simulink model "SixDof"  (R2023a)
settings: Solver=VariableStepAuto  StartTime=0.0  StopTime=60  RelTol=1e-3
values from neighbouring files (symbols this model uses):
  b = 9.144    [FS.m]
  c = 3.45    [FS.m]
  delta_r = 0    [FS.m]
  deltalef = 0    [FS.m]
  deltaSB = 0    [FS.m]
  F16_LookupTables =     [F16_LookupTables.mat]
  g = 9.80665    [FS.m]
  Ixx = 12875    [FS.m]
  Ixz = 1331    [FS.m]
  Iyy = 75674    [FS.m]
  Izz = 85552    [FS.m]
  mass = 9300    [FS.m]
  S = 27.88    [FS.m]
undefined symbols (not defined in the file or in its folder): Earth, WGS84
libraries: coeff x6, simulink_extras x4, shared6dof x1, aerolibtransform2 x1, aerolibfltsims x1, AtmosferModel x1, aerolibasang x1, simulink x1, sharedtransform x1, propulsive x1, uavutilslib x1
(part 1 of 2)
settings Model: Creator=User  LastModifiedBy=User
settings SolverCC: ZeroCrossAlgorithm=Adaptive
settings DebuggingCC: MaskedZcDiagnostic=none  IgnoredZcDiagnostic=none

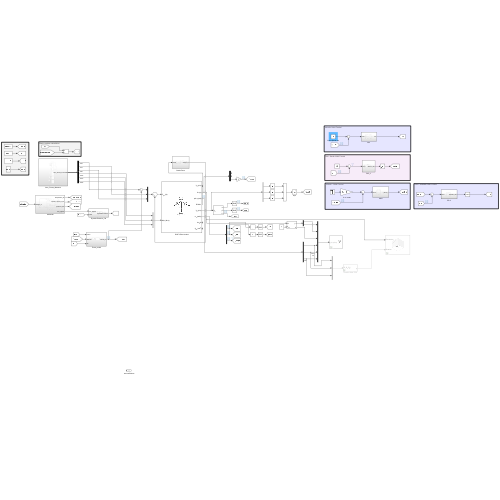
[thumbnail: Simulink's stored preview of the top-level diagram]
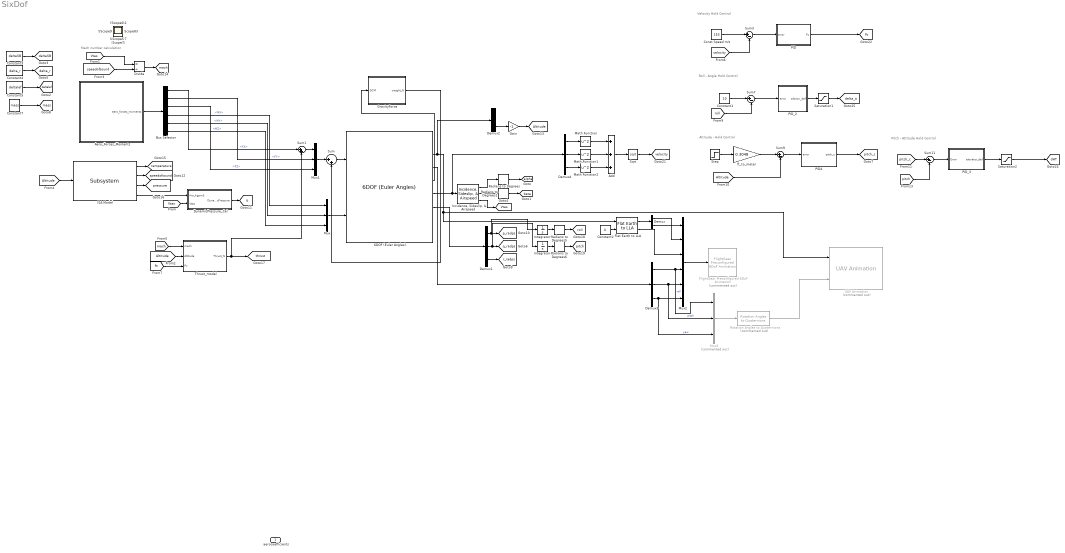
== system SixDof ==
  note: Altitude - Hold Control
  note: Pitch - Attitude Hold Control
  note: Roll - Angle Hold Control
  note: Velocity Hold Control
  note: Mach number calculation
  6DOF (Euler Angles) : shared6dof/6DOF (Euler Angles)  units=Metric (MKS)  mtype=Fixed  rep=Euler Angles  xme_0=[0 0 -3048]  Vm_0=[0 153 0]  eul_0=[0 0 0]  pm_0=[0 0 0]  mass_0=mass  mass_e=0.5  mass_f=2.0  inertia=[Ixx 0 Ixz; 0 Iyy 0; 0 0 Izz]  inertia_e=eye(3)  inertia_f=2*eye(3)  k_quat=1.0  vre_flag=on  abi_flag=off  aMode=0  xme_statename=''  Vm_statename=''  eul_statename=''  quat_statename=''  pm_statename=''  mass_statename=''
  Add : Sum  Inputs=+++
  Aero_Forces_Moments : Subsystem
  Bus Selector : BusSelector  OutputSignals=FX,FY,FZ,MX,MY,MZ
  Const Speed m/s : Constant  Value=153
  Constant1 : Constant  Value=10
  Constant2 : Constant  Value=0
  Constant3 : Constant  Value=deltaSB
  Constant4 : Constant  Value=delta_r
  Constant5 : Constant  Value=deltalef
  Constant7 : Constant  Value=mass
  Demux : Demux  Outputs=2
  Demux{1..4} (4 alike) : Demux  Outputs=3
  Divide : Product  Inputs=*/
  DynamicPressure_Cal : Subsystem
  Flat Earth to LLA : aerolibtransform2/Flat Earth to LLA  units=Metric (MKS)  ptype=Earth (WGS84)  F=1/298.257223563  R=6378137  refPosPort=off  LL0=[0 10]  psi=0
  FlightGear Preconfigured 6DoF Animation : aerolibfltsims/FlightGear Preconfigured 6DoF Animation  Commented=on  xFlightGearVersion=v2019.1  DestinationIpAddress=127.0.0.1  DestinationPort=5502  SampleTime=1/30  packetVersion=24
  Gain : Gain  Gain=-1
  GravityForce : Subsystem
  ISA Model : AtmosferModel/Subsystem  SystemSampleTime=-1  VariantActivationTime=update diagram  Latency=0  AutoFrameSizeCalculation=off
  "Incidence, Sideslip, & Airspeed" : aerolibasang/Incidence, Sideslip, & Airspeed
  Integrator2 : Integrator
  Integrator4 : Integrator
  Math Function : Math  Operator=square
  Math Function1 : Math  Operator=square
  Math Function2 : Math  Operator=square
  Mux : Mux  Inputs=3
  Mux1 : Mux  Inputs=3
  Mux2 : Mux  Inputs=6
  Mux3 : Mux  Commented=on  Inputs=3
  "PID " : Subsystem
  PID4 : Subsystem
  PID_2 : Subsystem
  PID_3 : Subsystem
  Radians to Degrees{,1,5..6} (4 alike) : simulink_extras/Transformations/Radians to Degrees
  Rotation Angles to Quaternions : sharedtransform/Rotation Angles to Quaternions  Commented=on  rotationOrder=ZYX  aMode=aMode
  Saturation1 : Saturate  UpperLimit=20  LowerLimit=-20
  Saturation2 : Saturate  UpperLimit=20  LowerLimit=-20  LinearizeAsGain=off  ZeroCross=off
  Sqrt : Sqrt  IntermediateResultsDataTypeStr=double
  Step : Step  Time=30  Before=11000  After=9900  SampleTime=0
  Sum : Sum  Inputs=|++
  Sum1 : Sum  Inputs=|++
  Sum{3,7,9,11} (4 alike) : Sum  Inputs=|+-
  Thrust_model : Subsystem
  UAV Animation : uavutilslib/UAV Animation  Commented=on  UAVType=FixedWing  UAVSize=1  InertialZDirection=Down  SampleTime=-1
  ft_to_meter : Gain  Gain=0.3048
  aerocoefficients : Outport
  Scope{,1..44} (45 alike) : Scope
  tag scope: Altitude=global, Pc=global, Vtas=global, alpha=global, beta=global, dHT=global, deltaSB=global, delta_a=global, delta_r=global, deltalef=global, mach=global, mass=global, p_radps=global, pitch=global, pitch_c=global, pressure=global, q=global, q_radps=global, r_radps=global, roll=global, speedofsound=global, temperature=global, thrust=global, velocity=global
  wires:
  [speedofsound] -> Divide/2
  [Vtas] -> Divide/1
  Demux1/1 -> Integrator2/1, [p_radps]
  Demux1/2 -> Integrator4/1, [q_radps]
  Demux1/3 -> [r_radps]
  6DOF (Euler Angles)/6 -> Demux1/1
  Aero_Forces_Moments/1(aero_forces_moments) -> Bus Selector/1
  Mux/1 -> 6DOF (Euler Angles)/2
  Constant3/1 -> [deltaSB]
  Constant4/1 -> [delta_r]
  Constant5/1 -> [deltalef]
  Constant7/1 -> [mass]
  6DOF (Euler Angles)/5 -> Demux4/1, "Incidence, Sideslip, & Airspeed"/1
  "Incidence, Sideslip, & Airspeed"/1 -> Radians to Degrees/1
  "Incidence, Sideslip, & Airspeed"/2 -> Radians to Degrees1/1
  "Incidence, Sideslip, & Airspeed"/3 -> [Vtas]
  Bus Selector/2 -> Mux1/2  "<FY>"
  Bus Selector/4 -> Mux/1  "<MX>"
  Bus Selector/5 -> Mux/2  "<MY>"
  Bus Selector/6 -> Mux/3  "<MZ>"
  Bus Selector/3 -> Mux1/3  "<FZ>"
  Mux1/1 -> Sum/1
  Sum/1 -> 6DOF (Euler Angles)/1
  6DOF (Euler Angles)/2 -> Demux2/1, Flat Earth to LLA/1, UAV Animation/1
  Radians to Degrees1/1 -> [beta]
  Radians to Degrees/1 -> [alpha]
  6DOF (Euler Angles)/4 -> GravityForce/1(DCM)
  GravityForce/1(weight_N) -> Sum/2
  DynamicPressure_Cal/1(DynamicPressure) -> [q]
  [Vtas] -> DynamicPressure_Cal/2(Vtas)
  Divide/1 -> [mach]
  Sum1/1 -> Mux1/1
  Bus Selector/1 -> Sum1/1  "<FX>"
  Thrust_model/1(Thrust_N) -> Sum1/2, [thrust]
  [mach] -> Thrust_model/1(mach)
  [Altitude] -> Thrust_model/2(Altitude)
  [Altitude] -> ISA Model/1
  ISA Model/3 -> [pressure]
  ISA Model/2 -> [speedofsound]
  ISA Model/1 -> [temperature]
  ISA Model/4 -> DynamicPressure_Cal/1(rho_kgpm3)
  Gain/1 -> [Altitude]
  6DOF (Euler Angles)/3 -> Demux3/1
  Demux4/1 -> Math Function/1
  Demux4/3 -> Math Function2/1
  Demux4/2 -> Math Function1/1
  Math Function/1 -> Add/1
  Math Function1/1 -> Add/2
  Math Function2/1 -> Add/3
  Add/1 -> Sqrt/1
  Sqrt/1 -> [velocity]
  [velocity] -> Sum3/2
  Const Speed m/s/1 -> Sum3/1
  [Pc] -> Thrust_model/3(Pc)
  [roll] -> Sum7/2
  Integrator2/1 -> Radians to Degrees5/1
  Radians to Degrees5/1 -> [roll]
  Integrator4/1 -> Radians to Degrees6/1
  Radians to Degrees6/1 -> [pitch]
  [Altitude] -> Sum9/2
  [pitch] -> Sum11/2
  Sum3/1 -> "PID "/1(error)
  "PID "/1(Pc) -> [Pc]
  Sum7/1 -> PID_2/1(error)
  PID_2/1(aileron_def) -> Saturation1/1
  Sum11/1 -> PID_3/1(Error)
  PID_3/1(elevator_def) -> Saturation2/1
  Saturation1/1 -> [delta_a]
  Mux2/1 -> FlightGear Preconfigured 6DoF Animation/1
  Flat Earth to LLA/1 -> Demux/1
  Demux/2 -> Mux2/1
  Demux/1 -> Mux2/2
  Constant2/1 -> Flat Earth to LLA/2
  Flat Earth to LLA/2 -> Mux2/3
  Demux3/1 -> Mux3/1, Mux2/4  "roll"
  Demux3/2 -> Mux3/2, Mux2/5  "pitch"
  Demux3/3 -> Mux3/3, Mux2/6  "yaw"
  Constant1/1 -> Sum7/1
  Step/1 -> ft_to_meter/1
  ft_to_meter/1 -> Sum9/1
  Saturation2/1 -> [dHT]
  Rotation Angles to Quaternions/1 -> UAV Animation/2
  Mux3/1 -> Rotation Angles to Quaternions/1
  [pitch_c] -> Sum11/1
  Demux2/3 -> Gain/1
  Sum9/1 -> PID4/1(error)
  PID4/1(pitch_c) -> [pitch_c]

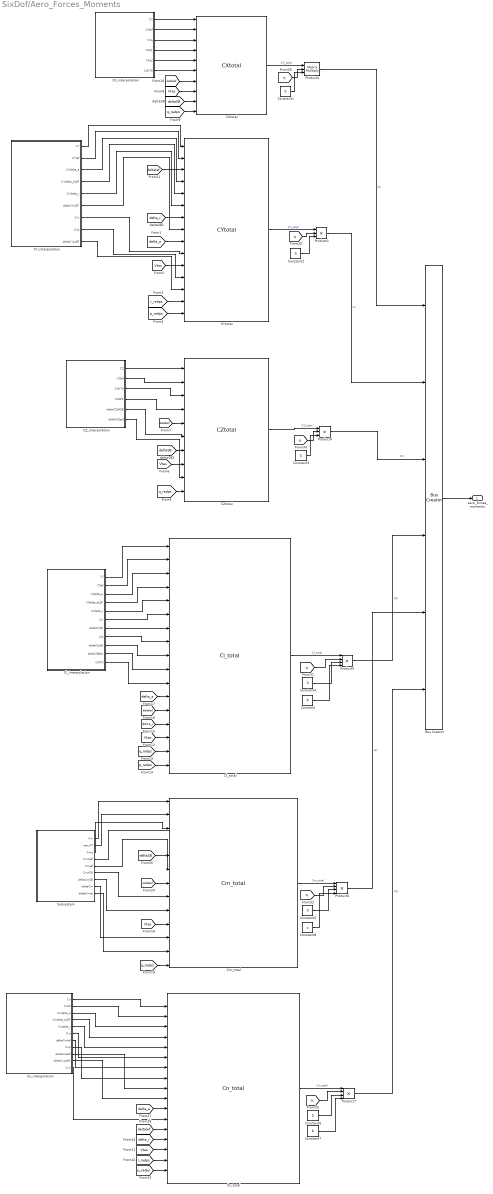
== system SixDof/Aero_Forces_Moments ==
  Bus Creator : BusCreator  Inputs=6
  CX_interpolation : Subsystem
  CXtotal : coeff/CXtotal  SystemSampleTime=-1  VariantActivationTime=update diagram  Latency=0  AutoFrameSizeCalculation=off
  CY_interpolation : Subsystem
  CYtotal : coeff/CYtotal  SystemSampleTime=-1  VariantActivationTime=update diagram  Latency=0  AutoFrameSizeCalculation=off
  CZ_interpolation : Subsystem
  CZtotal : coeff/CZtotal  SystemSampleTime=-1  VariantActivationTime=update diagram  Latency=0  AutoFrameSizeCalculation=off
  Cl_interpolation : Subsystem
  Cl_total : coeff/Cl_total  SystemSampleTime=-1  VariantActivationTime=update diagram  Latency=0  AutoFrameSizeCalculation=off
  Cm_total : coeff/Cm_total  SystemSampleTime=-1  VariantActivationTime=update diagram  Latency=0  AutoFrameSizeCalculation=off
  Cn_interpolation : Subsystem
  Cn_total : coeff/Cn_total  SystemSampleTime=-1  VariantActivationTime=update diagram  Latency=0  AutoFrameSizeCalculation=off
  Constant : Constant  Value=b
  Constant{1..6} (6 alike) : Constant  Value=S
  Constant7 : Constant  Value=b
  Constant8 : Constant  Value=c
  Product2 : Product  Inputs=3  Multiplication=Matrix(*)
  Product3 : Product  Inputs=3
  Product4 : Product  Inputs=3
  Product5 : Product  Inputs=4
  Product6 : Product  Inputs=4
  Product7 : Product  Inputs=4
  Subsystem : Subsystem
  aero_forces_moments : Outport
  wires:
  [p_radps] -> Cl_total/17
  CY_interpolation/3(CYdelta_a) -> CYtotal/4
  Cn_interpolation/9(deltaCnplef) -> Cn_total/9
  Subsystem/9(deltaCmds) -> Cm_total/12
  CZ_interpolation/1(CZ) -> CZtotal/1
  [deltalef] -> Cl_total/13
  [Vtas] -> Cm_total/10
  CX_interpolation/4(CXq1) -> CXtotal/4
  [deltalef] -> CXtotal/7
  [Vtas] -> CXtotal/8
  [p_radps] -> CYtotal/15
  Cl_interpolation/2(Cllef) -> Cl_total/2
  CZ_interpolation/5(deltaCZlefSB) -> CZtotal/6
  Cl_interpolation/4(Cldelta_aLEF) -> Cl_total/4
  Cl_interpolation/3(Cldelta_a) -> Cl_total/3
  CX_interpolation/1(CX) -> CXtotal/1
  Subsystem/4(Cmqlef) -> Cm_total/4
  CX_interpolation/2(CXlef) -> CXtotal/2
  CY_interpolation/8(CYp) -> CYtotal/12
  [Vtas] -> Cn_total/15
  Subsystem/3(Cmq) -> Cm_total/3
  Cl_interpolation/10(deltaClBeta) -> Cl_total/10
  Subsystem/7(deltaCmSB) -> Cm_total/9
  CX_interpolation/3(CXq) -> CXtotal/3
  Cn_interpolation/2(Cnlef) -> Cn_total/2
  [deltaSB] -> CXtotal/9
  CZ_interpolation/4(CZlef1) -> CZtotal/4
  CY_interpolation/1(CY) -> CYtotal/1
  CX_interpolation/5(CXq2) -> CXtotal/5
  CX_interpolation/6(CXHT0) -> CXtotal/6
  [r_radps] -> Cn_total/16
  Subsystem/5(Cmlef) -> Cm_total/6
  CY_interpolation/2(CYlef) -> CYtotal/2
  CY_interpolation/4(CYdelta_aLEF) -> CYtotal/5
  [q_radps] -> Cl_total/16
  CZ_interpolation/3(CZHT0) -> CZtotal/3
  [deltalef] -> CYtotal/3
  Cn_interpolation/3(Cndelta_a) -> Cn_total/3
  [Vtas] -> CYtotal/11
  Subsystem/8(deltaCm) -> Cm_total/11
  Cl_interpolation/9(deltaClplef) -> Cl_total/9
  [delta_a] -> CYtotal/9
  Cl_interpolation/6(Clr) -> Cl_total/6
  [deltaSB] -> CZtotal/7
  CY_interpolation/6(deltaCYrLEF) -> CYtotal/8
  CZ_interpolation/2(CZlef) -> CZtotal/2
  [deltalef] -> Cm_total/7
  [delta_r] -> CYtotal/7
  Cl_interpolation/7(deltaClrlef) -> Cl_total/7
  CY_interpolation/9(deltaCYpLEF) -> CYtotal/13
  CZ_interpolation/6(deltaCZlqef) -> CZtotal/9
  [Vtas] -> CZtotal/8
  [Vtas] -> Cl_total/15
  Cn_interpolation/7(deltaCnrlef) -> Cn_total/7
  Subsystem/1(Cm) -> Cm_total/1
  Cl_interpolation/11(ClHT0) -> Cl_total/11
  [r_radps] -> CYtotal/14
  Cl_interpolation/8(Clp) -> Cl_total/8
  [q_radps] -> CZtotal/10
  [deltaSB] -> Cm_total/5
  Cl_interpolation/1(Cl) -> Cl_total/1
  [p_radps] -> Cn_total/17
  [q_radps] -> Cm_total/13
  Subsystem/6(CmHT0) -> Cm_total/8
  Cn_interpolation/6(Cnr) -> Cn_total/6
  Cn_interpolation/1(Cn) -> Cn_total/1
  CY_interpolation/7(CYr) -> CYtotal/10
  [deltalef] -> CZtotal/5
  Cn_interpolation/5(Cndelta_r) -> Cn_total/5
  Cn_interpolation/8(Cnp) -> Cn_total/8
  CY_interpolation/5(CYdelta_r) -> CYtotal/6
  Subsystem/2(eta_HT) -> Cm_total/2
  [q_radps] -> CXtotal/10
  Cl_interpolation/5(Cldelta_r) -> Cl_total/5
  Cn_interpolation/11(Cn1) -> Cn_total/12
  Cn_interpolation/4(Cndelta_aLEF) -> Cn_total/4
  [deltalef] -> Cn_total/13
  Cn_interpolation/10(deltaCnplef1) -> Cn_total/10
  Constant1/1 -> Product2/3
  [q] -> Product2/2
  CXtotal/1 -> Product2/1  "CX_total"
  Constant2/1 -> Product3/3
  [q] -> Product3/2
  CYtotal/1 -> Product3/1  "CY_total"
  Constant3/1 -> Product4/3
  [q] -> Product4/2
  CZtotal/1 -> Product4/1  "CZ_total"
  Constant4/1 -> Product5/3
  [q] -> Product5/2
  Cl_total/1 -> Product5/1  "Cl_total"
  Constant5/1 -> Product6/3
  [q] -> Product6/2
  Cm_total/1 -> Product6/1  "Cm_total"
  Constant6/1 -> Product7/3
  [q] -> Product7/2
  Cn_total/1 -> Product7/1  "Cn_total"
  Product2/1 -> Bus Creator/1  "FX"
  Product3/1 -> Bus Creator/2  "FY"
  Product4/1 -> Bus Creator/3  "FZ"
  Product5/1 -> Bus Creator/4  "MX"
  Product6/1 -> Bus Creator/5  "MY"
  Product7/1 -> Bus Creator/6  "MZ"
  Bus Creator/1 -> aero_forces_moments/1
  Constant/1 -> Product5/4
  Constant8/1 -> Product6/4
  Constant7/1 -> Product7/4
  [delta_a] -> Cl_total/12
  [delta_r] -> Cl_total/14
  [delta_a] -> Cn_total/11
  [delta_r] -> Cn_total/14

== system SixDof/DynamicPressure_Cal ==
  rho_kgpm3 : Inport
  Vtas : Inport  Port=2
  Gain : Gain  Gain=0.5
  Math Function : Math  Operator=square
  Product : Product
  DynamicPressure : Outport
  wires:
  Math Function/1 -> Gain/1
  Gain/1 -> Product/1
  rho_kgpm3/1 -> Product/2
  Product/1 -> DynamicPressure/1
  Vtas/1 -> Math Function/1

== system SixDof/GravityForce ==
  DCM : Inport
  Constant1 : Constant  Value=0
  Mux2 : Mux  Inputs=3
  Product1 : Product  Multiplication=Matrix(*)
  g_mps2 : Gain  Gain=g
  weight_N : Outport
  wires:
  Constant1/1 -> Mux2/1, Mux2/2
  Mux2/1 -> Product1/2
  g_mps2/1 -> Mux2/3  "weight_N"
  [mass] -> g_mps2/1
  Product1/1 -> weight_N/1  "weight_N"
  DCM/1 -> Product1/1

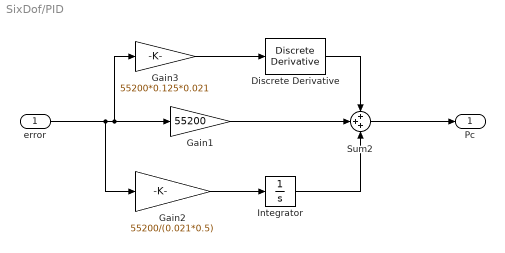
== system SixDof/PID  ==
  error : Inport
  Discrete Derivative : simulink/Discrete/Discrete Derivative  gainval=1.0  ICPrevScaledInput=0.0  OutMin=[]  OutMax=[]  OutDataType=fixdt(1, 16)  OutScaling=2^-10  DoSatur=off
  Gain1 : Gain  Gain=55200
  Gain2 : Gain  Gain=55200/(0.021*0.5)
  Gain3 : Gain  Gain=55200*0.125*0.021
  Integrator : Integrator
  Sum2 : Sum  Inputs=+++
  Pc : Outport
  wires:
  Gain3/1 -> Discrete Derivative/1
  Discrete Derivative/1 -> Sum2/1
  Integrator/1 -> Sum2/3
  Gain2/1 -> Integrator/1
  error/1 -> Gain2/1, Gain3/1, Gain1/1
  Gain1/1 -> Sum2/2
  Sum2/1 -> Pc/1

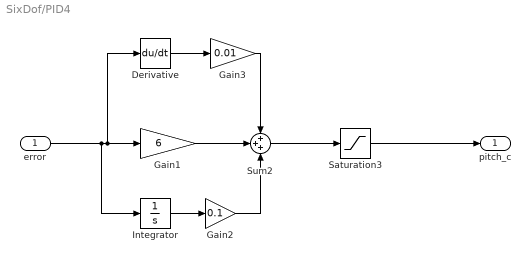
== system SixDof/PID4 ==
  error : Inport
  Derivative : Derivative
  Gain1 : Gain  Gain=6
  Gain2 : Gain  Gain=0.1
  Gain3 : Gain  Gain=0.01
  Integrator : Integrator
  Saturation3 : Saturate  UpperLimit=5  LowerLimit=-5
  Sum2 : Sum  Inputs=+++
  pitch_c : Outport
  wires:
  Gain1/1 -> Sum2/2
  error/1 -> Integrator/1, Derivative/1, Gain1/1
  Gain3/1 -> Sum2/1
  Derivative/1 -> Gain3/1
  Integrator/1 -> Gain2/1
  Gain2/1 -> Sum2/3
  Sum2/1 -> Saturation3/1
  Saturation3/1 -> pitch_c/1

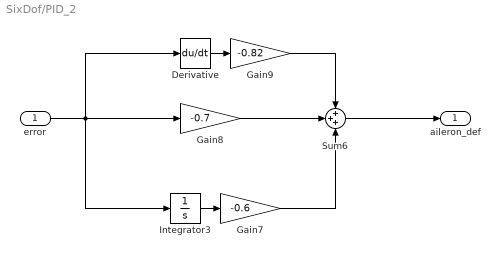
== system SixDof/PID_2 ==
  error : Inport
  Derivative : Derivative
  Gain7 : Gain  Gain=-0.6
  Gain8 : Gain  Gain=-0.7
  Gain9 : Gain  Gain=-0.82
  Integrator3 : Integrator
  Sum6 : Sum  Inputs=+++
  aileron_def : Outport
  wires:
  Gain7/1 -> Sum6/3
  error/1 -> Derivative/1, Integrator3/1, Gain8/1
  Gain8/1 -> Sum6/2
  Sum6/1 -> aileron_def/1
  Gain9/1 -> Sum6/1
  Integrator3/1 -> Gain7/1
  Derivative/1 -> Gain9/1

== system SixDof/PID_3 ==
  Error : Inport
  Derivative2 : Derivative
  Gain13 : Gain  Gain=-1.89
  Gain14 : Gain  Gain=-8
  Gain15 : Gain  Gain=-6
  Integrator6 : Integrator
  Sum10 : Sum  Inputs=+++
  elevator_def : Outport
  wires:
  Error/1 -> Integrator6/1, Derivative2/1, Gain14/1
  Gain15/1 -> Sum10/1
  Gain14/1 -> Sum10/2
  Derivative2/1 -> Gain15/1
  Integrator6/1 -> Gain13/1
  Gain13/1 -> Sum10/3
  Sum10/1 -> elevator_def/1

== system SixDof/Thrust_model ==
  mach : Inport
  Altitude : Inport  Port=2
  Pc : Inport  Port=3
  Propulsion : propulsive/Propulsive Force  SystemSampleTime=-1  VariantActivationTime=update diagram  Latency=0  AutoFrameSizeCalculation=off
  Thrust_interpolation : Subsystem
  ibstoN : Gain  Gain=4.4482216153
  meter_to_ft : Gain  Gain=3.28
  Thrust_N : Outport
  wires:
  ibstoN/1 -> Thrust_N/1
  Thrust_interpolation/3(max) -> Propulsion/3
  Thrust_interpolation/2(mil) -> Propulsion/2
  Thrust_interpolation/1(idle) -> Propulsion/1
  Propulsion/1 -> ibstoN/1
  meter_to_ft/1 -> Thrust_interpolation/2(altitude_ft)
  mach/1 -> Thrust_interpolation/1(mach)
  Altitude/1 -> meter_to_ft/1
  Pc/1 -> Propulsion/4

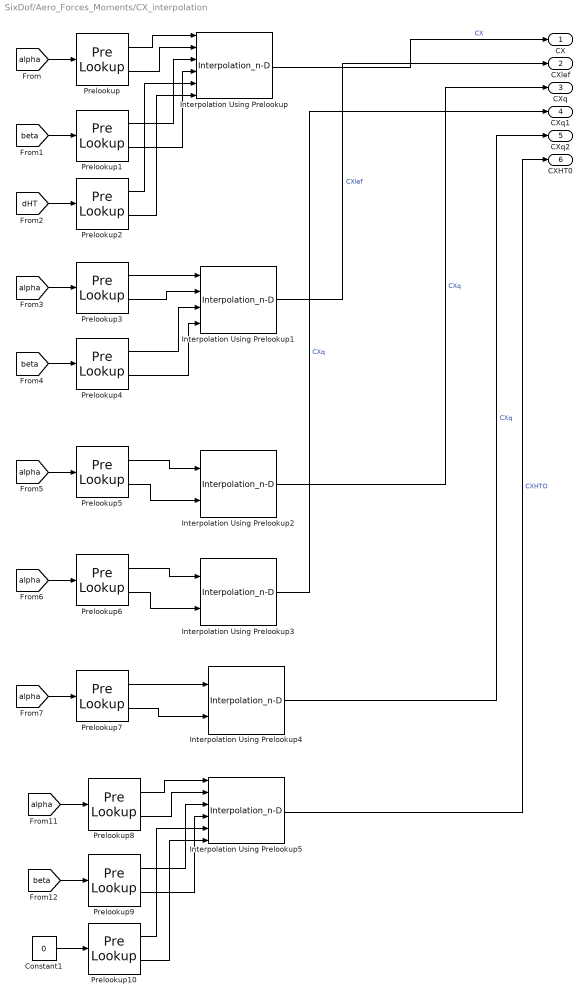
== system SixDof/Aero_Forces_Moments/CX_interpolation ==
  Constant1 : Constant  Value=0
  Interpolation Using Prelookup : Interpolation_n-D  NumberOfTableDimensions=3  Table=F16_LookupTables.aero.data.CX.CX  InternalRulePriority=Speed
      settings: InputPortMap=u0,u1,u2,u3,u4,u5
  Interpolation Using Prelookup1 : Interpolation_n-D  Table=F16_LookupTables.aero.data.CX.CXlef  InternalRulePriority=Speed
  Interpolation Using Prelookup2 : Interpolation_n-D  NumberOfTableDimensions=1  Table=F16_LookupTables.aero.data.CX.CXq  InternalRulePriority=Speed
      settings: InputPortMap=u0,u1
  Interpolation Using Prelookup3 : Interpolation_n-D  NumberOfTableDimensions=1  Table=F16_LookupTables.aero.data.CX.deltaCXqlef  InternalRulePriority=Speed
      settings: InputPortMap=u0,u1
  Interpolation Using Prelookup4 : Interpolation_n-D  NumberOfTableDimensions=1  Table=F16_LookupTables.aero.data.CX.deltaCXSB  InternalRulePriority=Speed
      settings: InputPortMap=u0,u1
  Interpolation Using Prelookup5 : Interpolation_n-D  NumberOfTableDimensions=3  Table=F16_LookupTables.aero.data.CX.CX  InternalRulePriority=Speed
      settings: InputPortMap=u0,u1,u2,u3,u4,u5
  Prelookup : PreLookup  BreakpointsData=F16_LookupTables.aero.inputs.CX.CX.alpha  ExtrapMethod=Linear
  Prelookup1 : PreLookup  BreakpointsData=F16_LookupTables.aero.inputs.CX.CX.beta  ExtrapMethod=Linear
  Prelookup10 : PreLookup  BreakpointsData=F16_LookupTables.aero.inputs.CX.CX.dHT  ExtrapMethod=Linear
  Prelookup2 : PreLookup  BreakpointsData=F16_LookupTables.aero.inputs.CX.CX.dHT  ExtrapMethod=Linear
  Prelookup3 : PreLookup  BreakpointsData=F16_LookupTables.aero.inputs.CX.CXlef.alpha  ExtrapMethod=Linear
  Prelookup4 : PreLookup  BreakpointsData=F16_LookupTables.aero.inputs.CX.CXlef.beta  ExtrapMethod=Linear
  Prelookup5 : PreLookup  BreakpointsData=F16_LookupTables.aero.inputs.CX.CXq.alpha  ExtrapMethod=Linear
  Prelookup6 : PreLookup  BreakpointsData=F16_LookupTables.aero.inputs.CX.deltaCXqlef.alpha  ExtrapMethod=Linear
  Prelookup7 : PreLookup  BreakpointsData=F16_LookupTables.aero.inputs.CX.deltaCXSB.alpha  ExtrapMethod=Linear
  Prelookup8 : PreLookup  BreakpointsData=F16_LookupTables.aero.inputs.CX.CX.alpha  ExtrapMethod=Linear
  Prelookup9 : PreLookup  BreakpointsData=F16_LookupTables.aero.inputs.CX.CX.beta  ExtrapMethod=Linear
  CX : Outport
  CXlef : Outport  Port=2
  CXq : Outport  Port=3
  CXq1 : Outport  Port=4
  CXq2 : Outport  Port=5
  CXHT0 : Outport  Port=6
  wires:
  [dHT] -> Prelookup2/1
  [beta] -> Prelookup9/1
  Prelookup4/1 -> Interpolation Using Prelookup1/3
  Constant1/1 -> Prelookup10/1
  Prelookup10/1 -> Interpolation Using Prelookup5/5
  [alpha] -> Prelookup3/1
  Prelookup1/1 -> Interpolation Using Prelookup/3
  [alpha] -> Prelookup5/1
  Prelookup10/2 -> Interpolation Using Prelookup5/6
  [alpha] -> Prelookup6/1
  Prelookup8/1 -> Interpolation Using Prelookup5/1
  Prelookup1/2 -> Interpolation Using Prelookup/4
  Interpolation Using Prelookup2/1 -> CXq/1  "CXq"
  [alpha] -> Prelookup8/1
  [beta] -> Prelookup4/1
  Interpolation Using Prelookup/1 -> CX/1  "CX"
  Interpolation Using Prelookup4/1 -> CXq2/1  "CXq"
  Prelookup9/2 -> Interpolation Using Prelookup5/4
  Prelookup/1 -> Interpolation Using Prelookup/1
  Prelookup/2 -> Interpolation Using Prelookup/2
  Prelookup3/1 -> Interpolation Using Prelookup1/1
  Prelookup4/2 -> Interpolation Using Prelookup1/4
  [alpha] -> Prelookup/1
  Prelookup5/2 -> Interpolation Using Prelookup2/2
  Prelookup3/2 -> Interpolation Using Prelookup1/2
  Prelookup2/1 -> Interpolation Using Prelookup/5
  Prelookup7/1 -> Interpolation Using Prelookup4/1
  [beta] -> Prelookup1/1
  Prelookup2/2 -> Interpolation Using Prelookup/6
  Prelookup9/1 -> Interpolation Using Prelookup5/3
  Prelookup6/2 -> Interpolation Using Prelookup3/2
  Prelookup6/1 -> Interpolation Using Prelookup3/1
  [alpha] -> Prelookup7/1
  Prelookup7/2 -> Interpolation Using Prelookup4/2
  Prelookup5/1 -> Interpolation Using Prelookup2/1
  Prelookup8/2 -> Interpolation Using Prelookup5/2
  Interpolation Using Prelookup1/1 -> CXlef/1  "CXlef"
  Interpolation Using Prelookup5/1 -> CXHT0/1  "CXHTO"
  Interpolation Using Prelookup3/1 -> CXq1/1  "CXq"

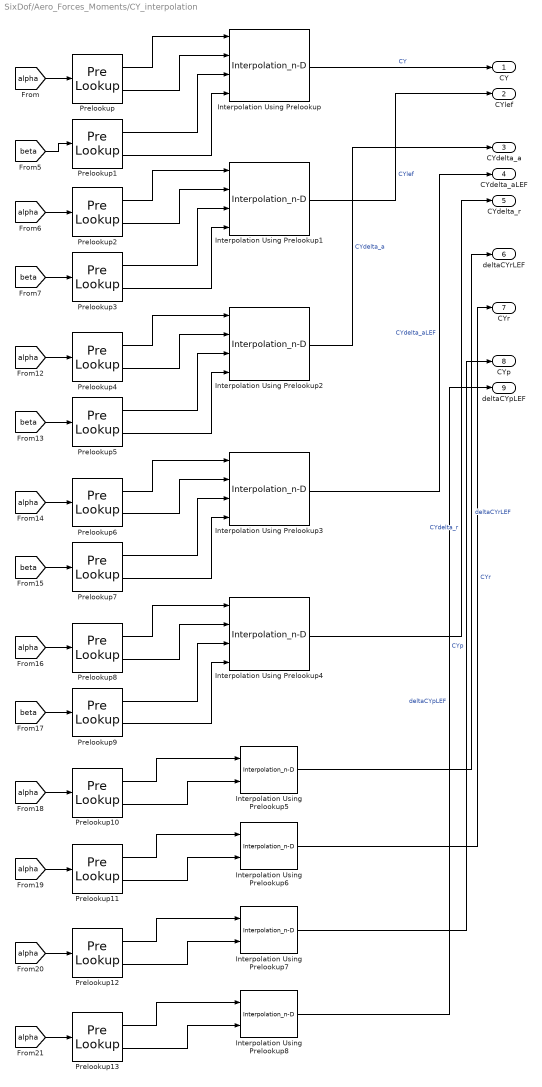
== system SixDof/Aero_Forces_Moments/CY_interpolation ==
  Interpolation Using Prelookup : Interpolation_n-D  Table=F16_LookupTables.aero.data.CY.CY  InternalRulePriority=Speed
  Interpolation Using Prelookup1 : Interpolation_n-D  Table=F16_LookupTables.aero.data.CY.CYlef  InternalRulePriority=Speed
  Interpolation Using Prelookup2 : Interpolation_n-D  Table=F16_LookupTables.aero.data.CY.CYdelta_a  InternalRulePriority=Speed
  Interpolation Using Prelookup3 : Interpolation_n-D  Table=F16_LookupTables.aero.data.CY.CYdelta_aLEF  InternalRulePriority=Speed
  Interpolation Using Prelookup4 : Interpolation_n-D  Table=F16_LookupTables.aero.data.CY.CYdelta_r  InternalRulePriority=Speed
  Interpolation Using Prelookup5 : Interpolation_n-D  NumberOfTableDimensions=1  Table=F16_LookupTables.aero.data.CY.deltaCYrlef  InternalRulePriority=Speed
      settings: InputPortMap=u0,u1
  Interpolation Using Prelookup6 : Interpolation_n-D  NumberOfTableDimensions=1  Table=F16_LookupTables.aero.data.CY.CYr  InternalRulePriority=Speed
      settings: InputPortMap=u0,u1
  Interpolation Using Prelookup7 : Interpolation_n-D  NumberOfTableDimensions=1  Table=F16_LookupTables.aero.data.CY.CYp  InternalRulePriority=Speed
      settings: InputPortMap=u0,u1
  Interpolation Using Prelookup8 : Interpolation_n-D  NumberOfTableDimensions=1  Table=F16_LookupTables.aero.data.CY.deltaCYplef  InternalRulePriority=Speed
      settings: InputPortMap=u0,u1
  Prelookup : PreLookup  BreakpointsData=F16_LookupTables.aero.inputs.CY.CY.alpha  ExtrapMethod=Linear
  Prelookup1 : PreLookup  BreakpointsData=F16_LookupTables.aero.inputs.CY.CY.beta  ExtrapMethod=Linear
  Prelookup10 : PreLookup  BreakpointsData=F16_LookupTables.aero.inputs.CY.deltaCYrlef.alpha  ExtrapMethod=Linear
  Prelookup11 : PreLookup  BreakpointsData=F16_LookupTables.aero.inputs.CY.CYr.alpha  ExtrapMethod=Linear
  Prelookup12 : PreLookup  BreakpointsData=F16_LookupTables.aero.inputs.CY.CYp.alpha  ExtrapMethod=Linear
  Prelookup13 : PreLookup  BreakpointsData=F16_LookupTables.aero.inputs.CY.deltaCYplef.alpha  ExtrapMethod=Linear
  Prelookup2 : PreLookup  BreakpointsData=F16_LookupTables.aero.inputs.CY.CYlef.alpha  ExtrapMethod=Linear
  Prelookup3 : PreLookup  BreakpointsData=F16_LookupTables.aero.inputs.CY.CYlef.beta  ExtrapMethod=Linear
  Prelookup4 : PreLookup  BreakpointsData=F16_LookupTables.aero.inputs.CY.CYdekta_a.alpha  ExtrapMethod=Linear
  Prelookup5 : PreLookup  BreakpointsData=F16_LookupTables.aero.inputs.CY.CYdekta_a.beta  ExtrapMethod=Linear
  Prelookup6 : PreLookup  BreakpointsData=F16_LookupTables.aero.inputs.CY.CYdelta_aLEF.alpha  ExtrapMethod=Linear
  Prelookup7 : PreLookup  BreakpointsData=F16_LookupTables.aero.inputs.CY.CYdelta_aLEF.beta  ExtrapMethod=Linear
  Prelookup8 : PreLookup  BreakpointsData=F16_LookupTables.aero.inputs.CY.CYdelta_r.alpha  ExtrapMethod=Linear
  Prelookup9 : PreLookup  BreakpointsData=F16_LookupTables.aero.inputs.CY.CYdelta_r.beta  ExtrapMethod=Linear
  CY : Outport
  CYlef : Outport  Port=2
  CYdelta_a : Outport  Port=3
  CYdelta_aLEF : Outport  Port=4
  CYdelta_r : Outport  Port=5
  deltaCYrLEF : Outport  Port=6
  CYr : Outport  Port=7
  CYp : Outport  Port=8
  deltaCYpLEF : Outport  Port=9
  wires:
  [alpha] -> Prelookup10/1
  [alpha] -> Prelookup13/1
  Prelookup2/2 -> Interpolation Using Prelookup1/2
  Interpolation Using Prelookup5/1 -> deltaCYrLEF/1  "deltaCYrLEF"
  Prelookup13/1 -> Interpolation Using Prelookup8/1
  Interpolation Using Prelookup6/1 -> CYr/1  "CYr"
  [alpha] -> Prelookup12/1
  Prelookup/1 -> Interpolation Using Prelookup/1
  Prelookup13/2 -> Interpolation Using Prelookup8/2
  Prelookup6/2 -> Interpolation Using Prelookup3/2
  [beta] -> Prelookup5/1
  [beta] -> Prelookup9/1
  [alpha] -> Prelookup/1
  Prelookup10/2 -> Interpolation Using Prelookup5/2
  Interpolation Using Prelookup/1 -> CY/1  "CY"
  Prelookup3/1 -> Interpolation Using Prelookup1/3
  [beta] -> Prelookup1/1
  Prelookup10/1 -> Interpolation Using Prelookup5/1
  Prelookup4/1 -> Interpolation Using Prelookup2/1
  Prelookup1/2 -> Interpolation Using Prelookup/4
  Prelookup6/1 -> Interpolation Using Prelookup3/1
  [beta] -> Prelookup3/1
  Prelookup8/1 -> Interpolation Using Prelookup4/1
  Prelookup12/1 -> Interpolation Using Prelookup7/1
  [alpha] -> Prelookup6/1
  Interpolation Using Prelookup2/1 -> CYdelta_a/1  "CYdelta_a"
  Prelookup11/2 -> Interpolation Using Prelookup6/2
  Prelookup3/2 -> Interpolation Using Prelookup1/4
  Prelookup7/1 -> Interpolation Using Prelookup3/3
  Interpolation Using Prelookup4/1 -> CYdelta_r/1  "CYdelta_r"
  [beta] -> Prelookup7/1
  Prelookup7/2 -> Interpolation Using Prelookup3/4
  Prelookup11/1 -> Interpolation Using Prelookup6/1
  Prelookup12/2 -> Interpolation Using Prelookup7/2
  Interpolation Using Prelookup7/1 -> CYp/1  "CYp"
  Prelookup1/1 -> Interpolation Using Prelookup/3
  [alpha] -> Prelookup8/1
  Prelookup/2 -> Interpolation Using Prelookup/2
  [alpha] -> Prelookup2/1
  [alpha] -> Prelookup11/1
  [alpha] -> Prelookup4/1
  Prelookup2/1 -> Interpolation Using Prelookup1/1
  Prelookup9/2 -> Interpolation Using Prelookup4/4
  Prelookup5/1 -> Interpolation Using Prelookup2/3
  Prelookup4/2 -> Interpolation Using Prelookup2/2
  Prelookup5/2 -> Interpolation Using Prelookup2/4
  Prelookup8/2 -> Interpolation Using Prelookup4/2
  Interpolation Using Prelookup3/1 -> CYdelta_aLEF/1  "CYdelta_aLEF"
  Prelookup9/1 -> Interpolation Using Prelookup4/3
  Interpolation Using Prelookup1/1 -> CYlef/1  "CYlef"
  Interpolation Using Prelookup8/1 -> deltaCYpLEF/1  "deltaCYpLEF"

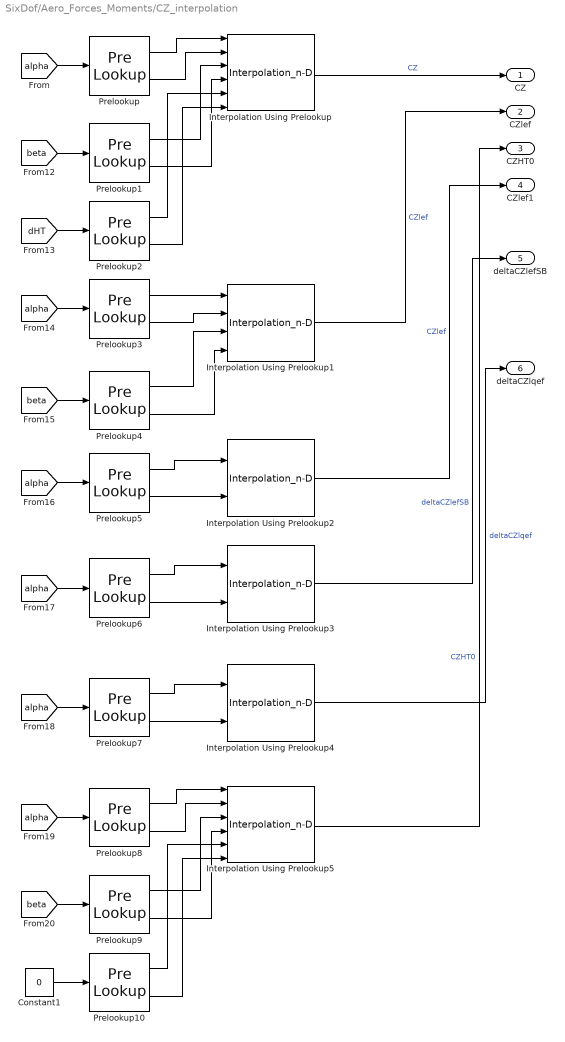
== system SixDof/Aero_Forces_Moments/CZ_interpolation ==
  Constant1 : Constant  Value=0
  Interpolation Using Prelookup : Interpolation_n-D  NumberOfTableDimensions=3  Table=F16_LookupTables.aero.data.CZ.CZ  InternalRulePriority=Speed
      settings: InputPortMap=u0,u1,u2,u3,u4,u5
  Interpolation Using Prelookup1 : Interpolation_n-D  Table=F16_LookupTables.aero.data.CZ.CZlef  InternalRulePriority=Speed
  Interpolation Using Prelookup2 : Interpolation_n-D  NumberOfTableDimensions=1  Table=F16_LookupTables.aero.data.CZ.CZq  InternalRulePriority=Speed
      settings: InputPortMap=u0,u1
  Interpolation Using Prelookup3 : Interpolation_n-D  NumberOfTableDimensions=1  Table=F16_LookupTables.aero.data.CZ.deltaCZSB  InternalRulePriority=Speed
      settings: InputPortMap=u0,u1
  Interpolation Using Prelookup4 : Interpolation_n-D  NumberOfTableDimensions=1  Table=F16_LookupTables.aero.data.CZ.deltaCZqlef  InternalRulePriority=Speed
      settings: InputPortMap=u0,u1
  Interpolation Using Prelookup5 : Interpolation_n-D  NumberOfTableDimensions=3  Table=F16_LookupTables.aero.data.CZ.CZ  InternalRulePriority=Speed
      settings: InputPortMap=u0,u1,u2,u3,u4,u5
  Prelookup : PreLookup  BreakpointsData=F16_LookupTables.aero.inputs.CZ.CZ.alpha  ExtrapMethod=Linear
  Prelookup1 : PreLookup  BreakpointsData=F16_LookupTables.aero.inputs.CZ.CZ.beta  ExtrapMethod=Linear
  Prelookup10 : PreLookup  BreakpointsData=F16_LookupTables.aero.inputs.CZ.CZ.dHT  ExtrapMethod=Linear
  Prelookup2 : PreLookup  BreakpointsData=F16_LookupTables.aero.inputs.CZ.CZ.dHT  ExtrapMethod=Linear
  Prelookup3 : PreLookup  BreakpointsData=F16_LookupTables.aero.inputs.CZ.CZlef.alpha  ExtrapMethod=Linear
  Prelookup4 : PreLookup  BreakpointsData=F16_LookupTables.aero.inputs.CZ.CZlef.beta  ExtrapMethod=Linear
  Prelookup5 : PreLookup  BreakpointsData=F16_LookupTables.aero.inputs.CZ.CZq.alpha  ExtrapMethod=Linear
  Prelookup6 : PreLookup  BreakpointsData=F16_LookupTables.aero.inputs.CZ.deltaCZSB.alpha  ExtrapMethod=Linear
  Prelookup7 : PreLookup  BreakpointsData=F16_LookupTables.aero.inputs.CZ.deltaCZqlef.alpha  ExtrapMethod=Linear
  Prelookup8 : PreLookup  BreakpointsData=F16_LookupTables.aero.inputs.CZ.CZ.alpha  ExtrapMethod=Linear
  Prelookup9 : PreLookup  BreakpointsData=F16_LookupTables.aero.inputs.CZ.CZ.beta  ExtrapMethod=Linear
  CZ : Outport
  CZlef : Outport  Port=2
  CZHT0 : Outport  Port=3
  CZlef1 : Outport  Port=4
  deltaCZlefSB : Outport  Port=5
  deltaCZlqef : Outport  Port=6
  wires:
  Prelookup9/1 -> Interpolation Using Prelookup5/3
  Prelookup/2 -> Interpolation Using Prelookup/2
  [beta] -> Prelookup9/1
  [alpha] -> Prelookup/1
  Prelookup6/1 -> Interpolation Using Prelookup3/1
  Prelookup10/1 -> Interpolation Using Prelookup5/5
  [alpha] -> Prelookup5/1
  Prelookup5/2 -> Interpolation Using Prelookup2/2
  Prelookup5/1 -> Interpolation Using Prelookup2/1
  Prelookup2/2 -> Interpolation Using Prelookup/6
  Prelookup8/2 -> Interpolation Using Prelookup5/2
  Prelookup8/1 -> Interpolation Using Prelookup5/1
  Prelookup2/1 -> Interpolation Using Prelookup/5
  Prelookup/1 -> Interpolation Using Prelookup/1
  Interpolation Using Prelookup2/1 -> CZlef1/1  "CZlef"
  Interpolation Using Prelookup/1 -> CZ/1  "CZ"
  [alpha] -> Prelookup8/1
  Prelookup6/2 -> Interpolation Using Prelookup3/2
  [alpha] -> Prelookup6/1
  [alpha] -> Prelookup7/1
  Prelookup1/2 -> Interpolation Using Prelookup/4
  Prelookup7/1 -> Interpolation Using Prelookup4/1
  Prelookup7/2 -> Interpolation Using Prelookup4/2
  [alpha] -> Prelookup3/1
  [dHT] -> Prelookup2/1
  [beta] -> Prelookup4/1
  Interpolation Using Prelookup5/1 -> CZHT0/1  "CZHT0"
  Prelookup3/2 -> Interpolation Using Prelookup1/2
  [beta] -> Prelookup1/1
  Prelookup4/1 -> Interpolation Using Prelookup1/3
  Prelookup3/1 -> Interpolation Using Prelookup1/1
  Prelookup1/1 -> Interpolation Using Prelookup/3
  Prelookup4/2 -> Interpolation Using Prelookup1/4
  Constant1/1 -> Prelookup10/1
  Prelookup10/2 -> Interpolation Using Prelookup5/6
  Prelookup9/2 -> Interpolation Using Prelookup5/4
  Interpolation Using Prelookup1/1 -> CZlef/1  "CZlef"
  Interpolation Using Prelookup4/1 -> deltaCZlqef/1  "deltaCZlqef"
  Interpolation Using Prelookup3/1 -> deltaCZlefSB/1  "deltaCZlefSB"

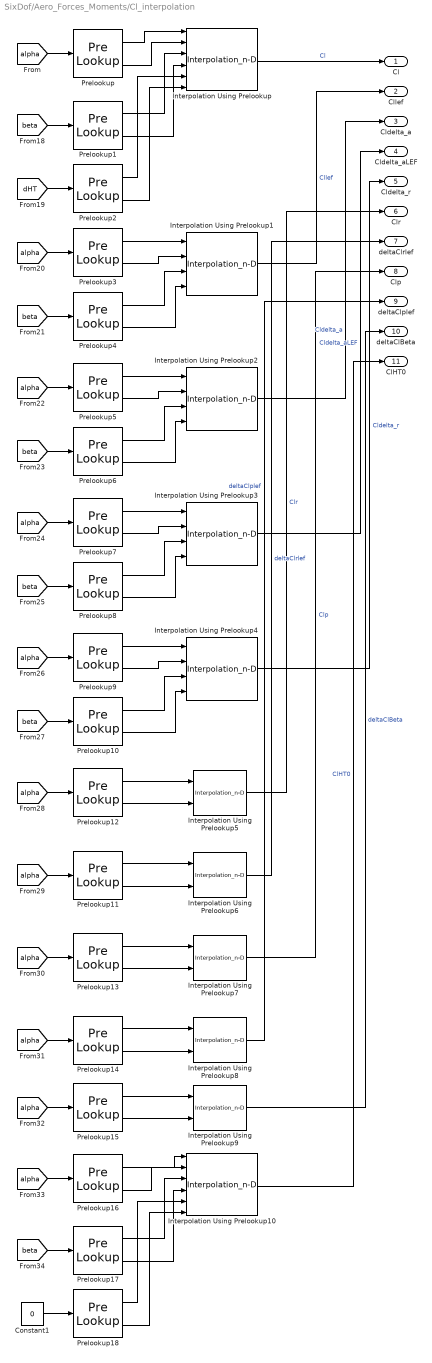
== system SixDof/Aero_Forces_Moments/Cl_interpolation ==
  Constant1 : Constant  Value=0
  Interpolation Using Prelookup : Interpolation_n-D  NumberOfTableDimensions=3  Table=F16_LookupTables.aero.data.Cl.Cl  InternalRulePriority=Speed
      settings: InputPortMap=u0,u1,u2,u3,u4,u5
  Interpolation Using Prelookup1 : Interpolation_n-D  Table=F16_LookupTables.aero.data.Cl.Cllef  InternalRulePriority=Speed
  Interpolation Using Prelookup10 : Interpolation_n-D  NumberOfTableDimensions=3  Table=F16_LookupTables.aero.data.Cl.Cl  InternalRulePriority=Speed
      settings: InputPortMap=u0,u1,u2,u3,u4,u5
  Interpolation Using Prelookup2 : Interpolation_n-D  Table=F16_LookupTables.aero.data.Cl.Cldelta_a  InternalRulePriority=Speed
  Interpolation Using Prelookup3 : Interpolation_n-D  Table=F16_LookupTables.aero.data.Cl.Cldelta_aLEF  InternalRulePriority=Speed
  Interpolation Using Prelookup4 : Interpolation_n-D  Table=F16_LookupTables.aero.data.Cl.Cldelta_r  InternalRulePriority=Speed
  Interpolation Using Prelookup5 : Interpolation_n-D  NumberOfTableDimensions=1  Table=F16_LookupTables.aero.data.Cl.Clr  InternalRulePriority=Speed
      settings: InputPortMap=u0,u1
  Interpolation Using Prelookup6 : Interpolation_n-D  NumberOfTableDimensions=1  Table=F16_LookupTables.aero.data.Cl.deltaClrlef  InternalRulePriority=Speed
      settings: InputPortMap=u0,u1
  Interpolation Using Prelookup7 : Interpolation_n-D  NumberOfTableDimensions=1  Table=F16_LookupTables.aero.data.Cl.Clp  InternalRulePriority=Speed
      settings: InputPortMap=u0,u1
  Interpolation Using Prelookup8 : Interpolation_n-D  NumberOfTableDimensions=1  Table=F16_LookupTables.aero.data.Cl.deltaClplef  InternalRulePriority=Speed
      settings: InputPortMap=u0,u1
  Interpolation Using Prelookup9 : Interpolation_n-D  NumberOfTableDimensions=1  Table=F16_LookupTables.aero.data.Cl.deltaClBeta  InternalRulePriority=Speed
      settings: InputPortMap=u0,u1
  Prelookup : PreLookup  BreakpointsData=F16_LookupTables.aero.inputs.Cl.Cl.alpha  ExtrapMethod=Linear
  Prelookup1 : PreLookup  BreakpointsData=F16_LookupTables.aero.inputs.Cl.Cl.beta  ExtrapMethod=Linear
  Prelookup10 : PreLookup  BreakpointsData=F16_LookupTables.aero.inputs.Cl.Cldelta_r.beta  ExtrapMethod=Linear
  Prelookup11 : PreLookup  BreakpointsData=F16_LookupTables.aero.inputs.Cl.deltaClrlef.alpha  ExtrapMethod=Linear
  Prelookup12 : PreLookup  BreakpointsData=F16_LookupTables.aero.inputs.Cl.Clr.alpha  ExtrapMethod=Linear
  Prelookup13 : PreLookup  BreakpointsData=F16_LookupTables.aero.inputs.Cl.Clp.alpha  ExtrapMethod=Linear
  Prelookup14 : PreLookup  BreakpointsData=F16_LookupTables.aero.inputs.Cl.deltaClplef.alpha  ExtrapMethod=Linear
  Prelookup15 : PreLookup  BreakpointsData=F16_LookupTables.aero.inputs.Cl.deltaClBeta.alpha  ExtrapMethod=Linear
  Prelookup16 : PreLookup  BreakpointsData=F16_LookupTables.aero.inputs.Cl.Cl.alpha  ExtrapMethod=Linear
  Prelookup17 : PreLookup  BreakpointsData=F16_LookupTables.aero.inputs.Cl.Cl.beta  ExtrapMethod=Linear
  Prelookup18 : PreLookup  BreakpointsData=F16_LookupTables.aero.inputs.Cl.Cl.dHT  ExtrapMethod=Linear
  Prelookup2 : PreLookup  BreakpointsData=F16_LookupTables.aero.inputs.Cl.Cl.dHT  ExtrapMethod=Linear
  Prelookup3 : PreLookup  BreakpointsData=F16_LookupTables.aero.inputs.Cl.Cllef.alpha  ExtrapMethod=Linear
  Prelookup4 : PreLookup  BreakpointsData=F16_LookupTables.aero.inputs.Cl.Cllef.beta  ExtrapMethod=Linear
  Prelookup5 : PreLookup  BreakpointsData=F16_LookupTables.aero.inputs.Cl.Cldelta_a.alpha  ExtrapMethod=Linear
  Prelookup6 : PreLookup  BreakpointsData=F16_LookupTables.aero.inputs.Cl.Cldelta_a.beta  ExtrapMethod=Linear
  Prelookup7 : PreLookup  BreakpointsData=F16_LookupTables.aero.inputs.Cl.Cldelta_aLEF.alpha  ExtrapMethod=Linear
  Prelookup8 : PreLookup  BreakpointsData=F16_LookupTables.aero.inputs.Cl.Cldelta_aLEF.beta  ExtrapMethod=Linear
  Prelookup9 : PreLookup  BreakpointsData=F16_LookupTables.aero.inputs.Cl.Cldelta_r.alpha  ExtrapMethod=Linear
  Cl : Outport
  Cllef : Outport  Port=2
  Cldelta_a : Outport  Port=3
  Cldelta_aLEF : Outport  Port=4
  Cldelta_r : Outport  Port=5
  Clr : Outport  Port=6
  deltaClrlef : Outport  Port=7
  Clp : Outport  Port=8
  deltaClplef : Outport  Port=9
  deltaClBeta : Outport  Port=10
  ClHT0 : Outport  Port=11
  wires:
  Prelookup2/1 -> Interpolation Using Prelookup/5
  Prelookup5/1 -> Interpolation Using Prelookup2/1
  Prelookup3/2 -> Interpolation Using Prelookup1/2
  Prelookup3/1 -> Interpolation Using Prelookup1/1
  Prelookup12/2 -> Interpolation Using Prelookup5/2
  Interpolation Using Prelookup/1 -> Cl/1  "Cl"
  Prelookup11/1 -> Interpolation Using Prelookup6/1
  Prelookup9/2 -> Interpolation Using Prelookup4/2
  [alpha] -> Prelookup3/1
  Prelookup4/2 -> Interpolation Using Prelookup1/4
  [beta] -> Prelookup6/1
  Interpolation Using Prelookup7/1 -> Clp/1  "Clp"
  [alpha] -> Prelookup11/1
  Prelookup9/1 -> Interpolation Using Prelookup4/1
  Prelookup5/2 -> Interpolation Using Prelookup2/2
  Prelookup18/1 -> Interpolation Using Prelookup10/5
  Prelookup6/1 -> Interpolation Using Prelookup2/3
  [dHT] -> Prelookup2/1
  Prelookup15/1 -> Interpolation Using Prelookup9/1
  [alpha] -> Prelookup12/1
  Prelookup6/2 -> Interpolation Using Prelookup2/4
  [alpha] -> Prelookup5/1
  Prelookup11/2 -> Interpolation Using Prelookup6/2
  [beta] -> Prelookup10/1
  [alpha] -> Prelookup13/1
  Interpolation Using Prelookup6/1 -> deltaClrlef/1  "deltaClrlef"
  Prelookup/2 -> Interpolation Using Prelookup/2
  [alpha] -> Prelookup15/1
  Prelookup13/1 -> Interpolation Using Prelookup7/1
  Prelookup17/2 -> Interpolation Using Prelookup10/4
  Prelookup16/2 -> Interpolation Using Prelookup10/2
  Prelookup16/1 -> Interpolation Using Prelookup10/1
  Prelookup15/2 -> Interpolation Using Prelookup9/2
  [alpha] -> Prelookup7/1
  Prelookup7/2 -> Interpolation Using Prelookup3/2
  [alpha] -> Prelookup/1
  Interpolation Using Prelookup10/1 -> ClHT0/1  "ClHT0"
  Prelookup7/1 -> Interpolation Using Prelookup3/1
  Prelookup8/2 -> Interpolation Using Prelookup3/4
  Interpolation Using Prelookup1/1 -> Cllef/1  "Cllef"
  Prelookup14/1 -> Interpolation Using Prelookup8/1
  [beta] -> Prelookup8/1
  [beta] -> Prelookup17/1
  Prelookup17/1 -> Interpolation Using Prelookup10/3
  [alpha] -> Prelookup14/1
  Prelookup1/2 -> Interpolation Using Prelookup/4
  Interpolation Using Prelookup3/1 -> Cldelta_aLEF/1  "Cldelta_aLEF"
  Prelookup8/1 -> Interpolation Using Prelookup3/3
  Prelookup1/1 -> Interpolation Using Prelookup/3
  Prelookup12/1 -> Interpolation Using Prelookup5/1
  [alpha] -> Prelookup16/1
  Prelookup/1 -> Interpolation Using Prelookup/1
  Prelookup4/1 -> Interpolation Using Prelookup1/3
  Prelookup2/2 -> Interpolation Using Prelookup/6
  [beta] -> Prelookup1/1
  Interpolation Using Prelookup9/1 -> deltaClBeta/1  "deltaClBeta"
  [beta] -> Prelookup4/1
  Prelookup18/2 -> Interpolation Using Prelookup10/6
  Prelookup10/2 -> Interpolation Using Prelookup4/4
  Prelookup10/1 -> Interpolation Using Prelookup4/3
  Prelookup14/2 -> Interpolation Using Prelookup8/2
  Constant1/1 -> Prelookup18/1
  [alpha] -> Prelookup9/1
  Prelookup13/2 -> Interpolation Using Prelookup7/2
  Interpolation Using Prelookup8/1 -> deltaClplef/1  "deltaClplef"
  Interpolation Using Prelookup2/1 -> Cldelta_a/1  "Cldelta_a"
  Interpolation Using Prelookup4/1 -> Cldelta_r/1  "Cldelta_r"
  Interpolation Using Prelookup5/1 -> Clr/1  "Clr"

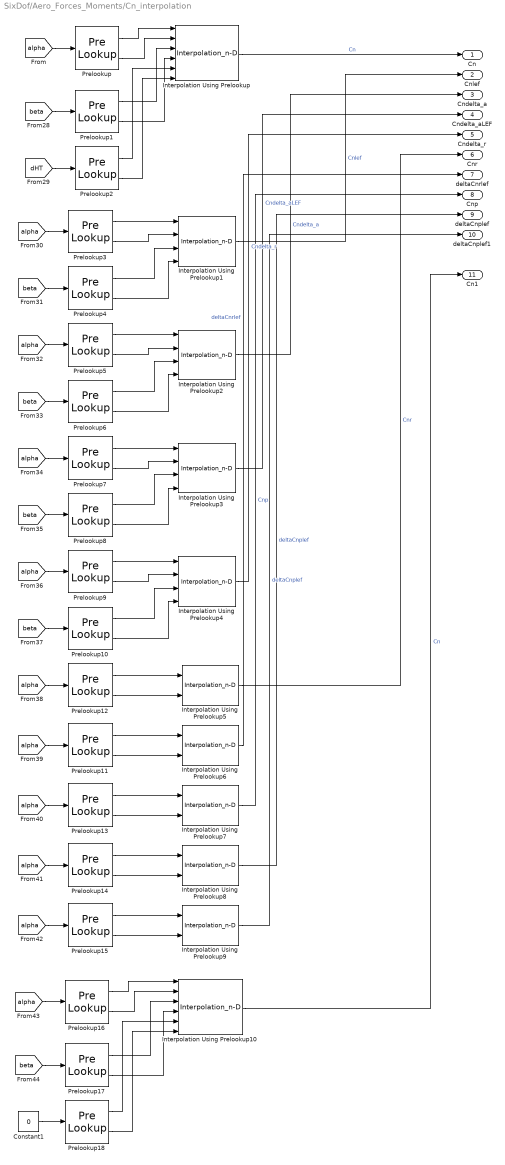
== system SixDof/Aero_Forces_Moments/Cn_interpolation ==
  Constant1 : Constant  Value=0
  Interpolation Using Prelookup : Interpolation_n-D  NumberOfTableDimensions=3  Table=F16_LookupTables.aero.data.Cn.Cn  InternalRulePriority=Speed
      settings: InputPortMap=u0,u1,u2,u3,u4,u5
  Interpolation Using Prelookup1 : Interpolation_n-D  Table=F16_LookupTables.aero.data.Cn.Cnlef  InternalRulePriority=Speed
  Interpolation Using Prelookup10 : Interpolation_n-D  NumberOfTableDimensions=3  Table=F16_LookupTables.aero.data.Cn.Cn  InternalRulePriority=Speed
      settings: InputPortMap=u0,u1,u2,u3,u4,u5
  Interpolation Using Prelookup2 : Interpolation_n-D  Table=F16_LookupTables.aero.data.Cn.Cndelta_a  InternalRulePriority=Speed
  Interpolation Using Prelookup3 : Interpolation_n-D  Table=F16_LookupTables.aero.data.Cn.Cndelta_aLEF  InternalRulePriority=Speed
  Interpolation Using Prelookup4 : Interpolation_n-D  Table=F16_LookupTables.aero.data.Cn.Cndelta_r  InternalRulePriority=Speed
  Interpolation Using Prelookup5 : Interpolation_n-D  NumberOfTableDimensions=1  Table=F16_LookupTables.aero.data.Cn.Cnr  InternalRulePriority=Speed
      settings: InputPortMap=u0,u1
  Interpolation Using Prelookup6 : Interpolation_n-D  NumberOfTableDimensions=1  Table=F16_LookupTables.aero.data.Cn.deltaCnrlef  InternalRulePriority=Speed
      settings: InputPortMap=u0,u1
  Interpolation Using Prelookup7 : Interpolation_n-D  NumberOfTableDimensions=1  Table=F16_LookupTables.aero.data.Cn.Cnp  InternalRulePriority=Speed
      settings: InputPortMap=u0,u1
  Interpolation Using Prelookup8 : Interpolation_n-D  NumberOfTableDimensions=1  Table=F16_LookupTables.aero.data.Cn.deltaCnplef  InternalRulePriority=Speed
      settings: InputPortMap=u0,u1
  Interpolation Using Prelookup9 : Interpolation_n-D  NumberOfTableDimensions=1  Table=F16_LookupTables.aero.data.Cn.deltaCnBeta  InternalRulePriority=Speed
      settings: InputPortMap=u0,u1
  Prelookup : PreLookup  BreakpointsData=F16_LookupTables.aero.inputs.Cn.Cn.alpha  ExtrapMethod=Linear
  Prelookup1 : PreLookup  BreakpointsData=F16_LookupTables.aero.inputs.Cn.Cn.beta  ExtrapMethod=Linear
  Prelookup10 : PreLookup  BreakpointsData=F16_LookupTables.aero.inputs.Cn.Cndelta_r.beta  ExtrapMethod=Linear
  Prelookup11 : PreLookup  BreakpointsData=F16_LookupTables.aero.inputs.Cn.deltaCnrlef.alpha  ExtrapMethod=Linear
  Prelookup12 : PreLookup  BreakpointsData=F16_LookupTables.aero.inputs.Cn.Cnr.alpha  ExtrapMethod=Linear
  Prelookup13 : PreLookup  BreakpointsData=F16_LookupTables.aero.inputs.Cn.Cnp.alpha  ExtrapMethod=Linear
  Prelookup14 : PreLookup  BreakpointsData=F16_LookupTables.aero.inputs.Cn.deltaCnplef.alpha  ExtrapMethod=Linear
  Prelookup15 : PreLookup  BreakpointsData=F16_LookupTables.aero.inputs.Cn.deltaCnBeta.alpha  ExtrapMethod=Linear
  Prelookup16 : PreLookup  BreakpointsData=F16_LookupTables.aero.inputs.Cn.Cn.alpha  ExtrapMethod=Linear
  Prelookup17 : PreLookup  BreakpointsData=F16_LookupTables.aero.inputs.Cn.Cn.beta  ExtrapMethod=Linear
  Prelookup18 : PreLookup  BreakpointsData=F16_LookupTables.aero.inputs.Cn.Cn.dHT  ExtrapMethod=Linear
  Prelookup2 : PreLookup  BreakpointsData=F16_LookupTables.aero.inputs.Cn.Cn.dHT  ExtrapMethod=Linear
  Prelookup3 : PreLookup  BreakpointsData=F16_LookupTables.aero.inputs.Cn.Cnlef.alpha  ExtrapMethod=Linear
  Prelookup4 : PreLookup  BreakpointsData=F16_LookupTables.aero.inputs.Cn.Cnlef.beta  ExtrapMethod=Linear
  Prelookup5 : PreLookup  BreakpointsData=F16_LookupTables.aero.inputs.Cn.Cndelta_a.alpha  ExtrapMethod=Linear
  Prelookup6 : PreLookup  BreakpointsData=F16_LookupTables.aero.inputs.Cn.Cndelta_a.beta  ExtrapMethod=Linear
  Prelookup7 : PreLookup  BreakpointsData=F16_LookupTables.aero.inputs.Cn.Cndelta_aLEF.alpha  ExtrapMethod=Linear
  Prelookup8 : PreLookup  BreakpointsData=F16_LookupTables.aero.inputs.Cn.Cndelta_aLEF.beta  ExtrapMethod=Linear
  Prelookup9 : PreLookup  BreakpointsData=F16_LookupTables.aero.inputs.Cn.Cndelta_r.alpha  ExtrapMethod=Linear
  Cn : Outport
  Cnlef : Outport  Port=2
  Cndelta_a : Outport  Port=3
  Cndelta_aLEF : Outport  Port=4
  Cndelta_r : Outport  Port=5
  Cnr : Outport  Port=6
  deltaCnrlef : Outport  Port=7
  Cnp : Outport  Port=8
  deltaCnplef : Outport  Port=9
  deltaCnplef1 : Outport  Port=10
  Cn1 : Outport  Port=11
  wires:
  Prelookup8/1 -> Interpolation Using Prelookup3/3
  Interpolation Using Prelookup4/1 -> Cndelta_r/1  "Cndelta_r"
  Prelookup17/1 -> Interpolation Using Prelookup10/3
  Prelookup15/1 -> Interpolation Using Prelookup9/1
  [alpha] -> Prelookup9/1
  [dHT] -> Prelookup2/1
  Prelookup7/1 -> Interpolation Using Prelookup3/1
  Interpolation Using Prelookup8/1 -> deltaCnplef/1  "deltaCnplef"
  Prelookup13/2 -> Interpolation Using Prelookup7/2
  Prelookup12/2 -> Interpolation Using Prelookup5/2
  Prelookup10/1 -> Interpolation Using Prelookup4/3
  Prelookup/1 -> Interpolation Using Prelookup/1
  Interpolation Using Prelookup2/1 -> Cndelta_a/1  "Cndelta_a"
  [alpha] -> Prelookup5/1
  Prelookup5/2 -> Interpolation Using Prelookup2/2
  Prelookup11/1 -> Interpolation Using Prelookup6/1
  Prelookup9/1 -> Interpolation Using Prelookup4/1
  Prelookup17/2 -> Interpolation Using Prelookup10/4
  Prelookup18/1 -> Interpolation Using Prelookup10/5
  Prelookup12/1 -> Interpolation Using Prelookup5/1
  [beta] -> Prelookup17/1
  [alpha] -> Prelookup12/1
  Prelookup6/1 -> Interpolation Using Prelookup2/3
  Prelookup13/1 -> Interpolation Using Prelookup7/1
  [beta] -> Prelookup4/1
  [alpha] -> Prelookup14/1
  [alpha] -> Prelookup13/1
  Prelookup/2 -> Interpolation Using Prelookup/2
  [beta] -> Prelookup1/1
  [beta] -> Prelookup8/1
  Prelookup3/1 -> Interpolation Using Prelookup1/1
  Interpolation Using Prelookup9/1 -> deltaCnplef1/1  "deltaCnplef"
  Prelookup3/2 -> Interpolation Using Prelookup1/2
  Prelookup4/2 -> Interpolation Using Prelookup1/4
  Prelookup4/1 -> Interpolation Using Prelookup1/3
  [alpha] -> Prelookup3/1
  [beta] -> Prelookup6/1
  Prelookup1/2 -> Interpolation Using Prelookup/4
  Prelookup1/1 -> Interpolation Using Prelookup/3
  Prelookup11/2 -> Interpolation Using Prelookup6/2
  Prelookup14/2 -> Interpolation Using Prelookup8/2
  [alpha] -> Prelookup15/1
  [alpha] -> Prelookup11/1
  [alpha] -> Prelookup16/1
  [alpha] -> Prelookup7/1
  Prelookup6/2 -> Interpolation Using Prelookup2/4
  Prelookup8/2 -> Interpolation Using Prelookup3/4
  Prelookup2/1 -> Interpolation Using Prelookup/5
  Prelookup7/2 -> Interpolation Using Prelookup3/2
  Prelookup16/2 -> Interpolation Using Prelookup10/2
  Interpolation Using Prelookup/1 -> Cn/1  "Cn"
  Constant1/1 -> Prelookup18/1
  Prelookup9/2 -> Interpolation Using Prelookup4/2
  [beta] -> Prelookup10/1
  Prelookup2/2 -> Interpolation Using Prelookup/6
  Prelookup10/2 -> Interpolation Using Prelookup4/4
  [alpha] -> Prelookup/1
  Prelookup14/1 -> Interpolation Using Prelookup8/1
  Interpolation Using Prelookup5/1 -> Cnr/1  "Cnr"
  Prelookup5/1 -> Interpolation Using Prelookup2/1
  Prelookup16/1 -> Interpolation Using Prelookup10/1
  Prelookup18/2 -> Interpolation Using Prelookup10/6
  Interpolation Using Prelookup7/1 -> Cnp/1  "Cnp"
  Prelookup15/2 -> Interpolation Using Prelookup9/2
  Interpolation Using Prelookup3/1 -> Cndelta_aLEF/1  "Cndelta_aLEF"
  Interpolation Using Prelookup1/1 -> Cnlef/1  "Cnlef"
  Interpolation Using Prelookup6/1 -> deltaCnrlef/1  "deltaCnrlef"
  Interpolation Using Prelookup10/1 -> Cn1/1  "Cn"
